simulink model "current_pi_model"  (R2023b)
settings: Solver=FixedStepDiscrete  StartTime=0.0  StopTime=current_pi_simcfg.stop_time  FixedStep=current_pi_simcfg.Ts_ctrl  RelTol=1e-3
values from neighbouring files (symbols this model uses):
  Kaw_id = 400.0    [current_pi_interface.sldd]
  Kaw_iq = 400.0    [current_pi_interface.sldd]
  Ki_id = 1072.4140625    [current_pi_interface.sldd]
  Ki_iq = 1072.4140625    [current_pi_interface.sldd]
  Kp_id = 1.3320353031158447    [current_pi_interface.sldd]
  Kp_iq = 1.3320353031158447    [current_pi_interface.sldd]
  VLimitRatio = 0.57700002193450928    [current_pi_interface.sldd]
undefined symbols (not defined in the file or in its folder): current_pi_simcfg, current_pi_test
settings Model: DataDictionary=current_pi_interface.sldd  Creator=user  LastModifiedBy=user
settings OptimizationCC: EnhancedBackFolding=on  PassReuseOutputArgsAs=Individual arguments  OptimizeBlockOrder=speed  DifferentSizesBufferReuse=on  OptimizationCustomize=off  EfficientTunableParamExpr=on
settings DebuggingCC: ParameterTunabilityLossMsg=error
settings HardwareCC: ProdBitPerPointer=32  ProdBitPerSizeT=32  ProdBitPerPtrDiffT=32  ProdLargestAtomicInteger=Long  ProdLargestAtomicFloat=Double  ProdWordSize=32  ProdHWDeviceType=ARM Compatible->ARM Cortex  TargetLargestAtomicInteger=Long  TargetLargestAtomicFloat=Double  TargetIntDivRoundTo=Zero  TargetEndianess=LittleEndian  TargetHWDeviceType=ARM Compatible->ARM Cortex  ProdEqTarget=off
settings SFSimCC: MATLABDynamicMemAlloc=off
settings RTWCC: Description=Embedded Coder  SystemTargetFile=ert.tlc  GenCodeOnly=on  TemplateMakefile=ert_default_tmf  GenerateReport=on
settings CodeAppCC: ForceParamTrailComments=on  IgnoreCustomStorageClasses=off  OperatorAnnotations=on  SimulinkDataObjDesc=on  SFDataObjDesc=on  InsertBlockDesc=on
settings ERTTargetCC: TargetLangStandard=C99 (ISO)  CodeInterfacePackaging=Reusable function  ERTCustomFileTemplate=example_file_process.tlc

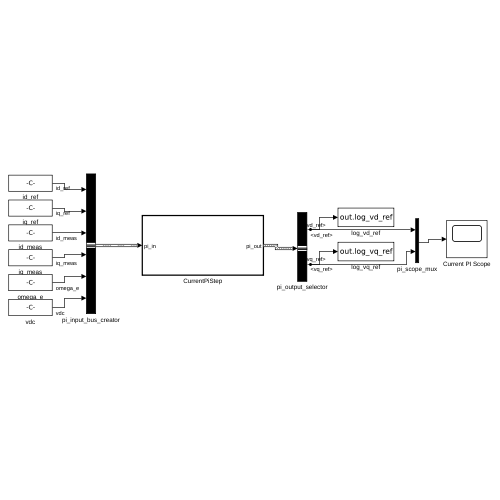
[thumbnail: Simulink's stored preview of the top-level diagram]
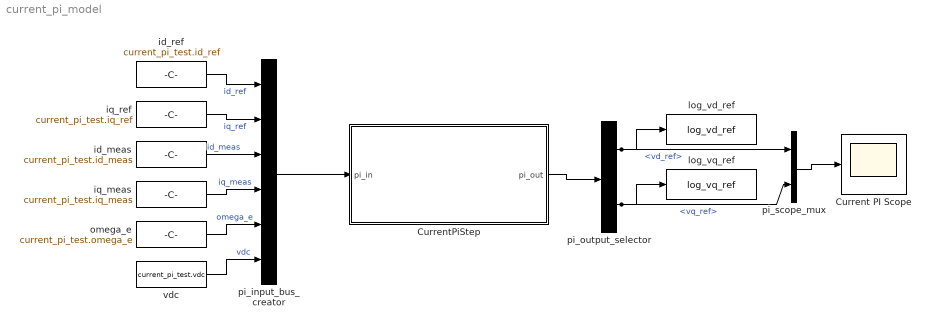
== system current_pi_model ==
  Current PI Scope : Scope
  CurrentPiStep : Subsystem  TreatAsAtomicUnit=on  RTWFcnName=CurrentPiStep  RTWFileName=CurrentPiStep
      settings: RTWFcnNameOpts=User specified  RTWFileNameOpts=User specified
  id_meas : Constant  Value=current_pi_test.id_meas  OutDataTypeStr=T_CurrentPiCurrent  SampleTime=current_pi_simcfg.Ts_ctrl
  id_ref : Constant  Value=current_pi_test.id_ref  OutDataTypeStr=T_CurrentPiCurrent  SampleTime=current_pi_simcfg.Ts_ctrl
  iq_meas : Constant  Value=current_pi_test.iq_meas  OutDataTypeStr=T_CurrentPiCurrent  SampleTime=current_pi_simcfg.Ts_ctrl
  iq_ref : Constant  Value=current_pi_test.iq_ref  OutDataTypeStr=T_CurrentPiCurrent  SampleTime=current_pi_simcfg.Ts_ctrl
  log_vd_ref : ToWorkspace  VariableName=log_vd_ref  SaveFormat=Timeseries  SampleTime=-1
  log_vq_ref : ToWorkspace  VariableName=log_vq_ref  SaveFormat=Timeseries  SampleTime=-1
  omega_e : Constant  Value=current_pi_test.omega_e  OutDataTypeStr=T_CurrentPiSpeed  SampleTime=current_pi_simcfg.Ts_ctrl
  pi_input_bus_creator : BusCreator  Inputs=6  OutDataTypeStr=Bus: current_pi_input_t  NonVirtualBus=on
  pi_output_selector : BusSelector  OutputSignals=vd_ref,vq_ref
  pi_scope_mux : Mux  Inputs=2
  vdc : Constant  Value=current_pi_test.vdc  OutDataTypeStr=T_CurrentPiVoltage  SampleTime=current_pi_simcfg.Ts_ctrl
  wires:
  id_ref/1 -> pi_input_bus_creator/1  "id_ref"
  iq_ref/1 -> pi_input_bus_creator/2  "iq_ref"
  id_meas/1 -> pi_input_bus_creator/3  "id_meas"
  iq_meas/1 -> pi_input_bus_creator/4  "iq_meas"
  omega_e/1 -> pi_input_bus_creator/5  "omega_e"
  vdc/1 -> pi_input_bus_creator/6  "vdc"
  pi_input_bus_creator/1 -> CurrentPiStep/1(pi_in)
  CurrentPiStep/1(pi_out) -> pi_output_selector/1
  pi_output_selector/1 -> log_vd_ref/1, pi_scope_mux/1  "<vd_ref>"
  pi_output_selector/2 -> log_vq_ref/1, pi_scope_mux/2  "<vq_ref>"
  pi_scope_mux/1 -> Current PI Scope/1

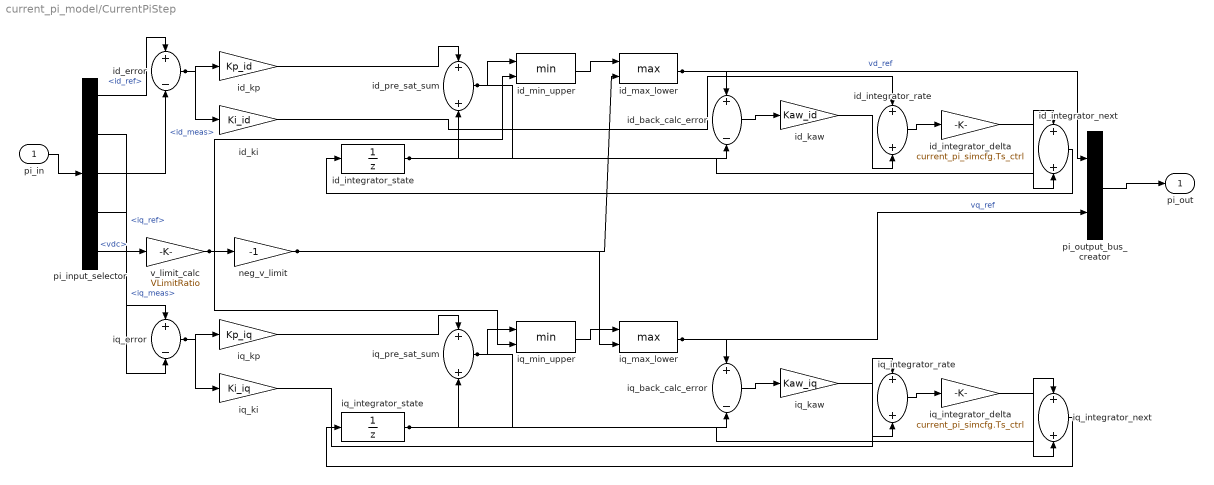
== system current_pi_model/CurrentPiStep ==
  pi_in : Inport  OutDataTypeStr=Bus: current_pi_input_t  BusOutputAsStruct=on
  id_back_calc_error : Sum  Inputs=+-  OutDataTypeStr=T_CurrentPiVoltage  AccumDataTypeStr=T_CurrentPiVoltage
  id_error : Sum  Inputs=+-  OutDataTypeStr=T_CurrentPiCurrent  AccumDataTypeStr=T_CurrentPiCurrent
  id_integrator_delta : Gain  Gain=current_pi_simcfg.Ts_ctrl  ParamDataTypeStr=T_CurrentPiFloat  OutDataTypeStr=T_CurrentPiVoltage
  id_integrator_next : Sum  OutDataTypeStr=T_CurrentPiVoltage  AccumDataTypeStr=T_CurrentPiVoltage
  id_integrator_rate : Sum  OutDataTypeStr=T_CurrentPiVoltage  AccumDataTypeStr=T_CurrentPiVoltage
  id_integrator_state : UnitDelay  SampleTime=current_pi_simcfg.Ts_ctrl  HasFrameUpgradeWarning=on
  id_kaw : Gain  Gain=Kaw_id  ParamDataTypeStr=T_CurrentPiGain  OutDataTypeStr=T_CurrentPiVoltage
  id_ki : Gain  Gain=Ki_id  ParamDataTypeStr=T_CurrentPiGain  OutDataTypeStr=T_CurrentPiVoltage
  id_kp : Gain  Gain=Kp_id  ParamDataTypeStr=T_CurrentPiGain  OutDataTypeStr=T_CurrentPiVoltage
  id_max_lower : MinMax  Function=max  Inputs=2
  id_min_upper : MinMax  Inputs=2
  id_pre_sat_sum : Sum  OutDataTypeStr=T_CurrentPiVoltage  AccumDataTypeStr=T_CurrentPiVoltage
  iq_back_calc_error : Sum  Inputs=+-  OutDataTypeStr=T_CurrentPiVoltage  AccumDataTypeStr=T_CurrentPiVoltage
  iq_error : Sum  Inputs=+-  OutDataTypeStr=T_CurrentPiCurrent  AccumDataTypeStr=T_CurrentPiCurrent
  iq_integrator_delta : Gain  Gain=current_pi_simcfg.Ts_ctrl  ParamDataTypeStr=T_CurrentPiFloat  OutDataTypeStr=T_CurrentPiVoltage
  iq_integrator_next : Sum  OutDataTypeStr=T_CurrentPiVoltage  AccumDataTypeStr=T_CurrentPiVoltage
  iq_integrator_rate : Sum  OutDataTypeStr=T_CurrentPiVoltage  AccumDataTypeStr=T_CurrentPiVoltage
  iq_integrator_state : UnitDelay  SampleTime=current_pi_simcfg.Ts_ctrl  HasFrameUpgradeWarning=on
  iq_kaw : Gain  Gain=Kaw_iq  ParamDataTypeStr=T_CurrentPiGain  OutDataTypeStr=T_CurrentPiVoltage
  iq_ki : Gain  Gain=Ki_iq  ParamDataTypeStr=T_CurrentPiGain  OutDataTypeStr=T_CurrentPiVoltage
  iq_kp : Gain  Gain=Kp_iq  ParamDataTypeStr=T_CurrentPiGain  OutDataTypeStr=T_CurrentPiVoltage
  iq_max_lower : MinMax  Function=max  Inputs=2
  iq_min_upper : MinMax  Inputs=2
  iq_pre_sat_sum : Sum  OutDataTypeStr=T_CurrentPiVoltage  AccumDataTypeStr=T_CurrentPiVoltage
  neg_v_limit : Gain  Gain=-1  ParamDataTypeStr=T_CurrentPiFloat  OutDataTypeStr=T_CurrentPiVoltage
  pi_input_selector : BusSelector  OutputSignals=id_ref,iq_ref,id_meas,iq_meas,vdc
  pi_output_bus_creator : BusCreator  Inputs=2  OutDataTypeStr=Bus: current_pi_output_t  NonVirtualBus=on
  v_limit_calc : Gain  Gain=VLimitRatio  ParamDataTypeStr=T_CurrentPiGain  OutDataTypeStr=T_CurrentPiVoltage
  pi_out : Outport  OutDataTypeStr=Bus: current_pi_output_t
  wires:
  pi_in/1 -> pi_input_selector/1
  pi_input_selector/5 -> v_limit_calc/1  "<vdc>"
  v_limit_calc/1 -> neg_v_limit/1, id_min_upper/2, iq_min_upper/2
  pi_input_selector/1 -> id_error/1  "<id_ref>"
  pi_input_selector/3 -> id_error/2  "<id_meas>"
  id_error/1 -> id_kp/1, id_ki/1
  id_kp/1 -> id_pre_sat_sum/1
  id_integrator_state/1 -> id_pre_sat_sum/2, id_integrator_next/1
  id_pre_sat_sum/1 -> id_min_upper/1, id_back_calc_error/2
  id_min_upper/1 -> id_max_lower/1
  neg_v_limit/1 -> id_max_lower/2, iq_max_lower/2
  id_max_lower/1 -> id_back_calc_error/1, pi_output_bus_creator/1  "vd_ref"
  id_back_calc_error/1 -> id_kaw/1
  id_ki/1 -> id_integrator_rate/1
  id_kaw/1 -> id_integrator_rate/2
  id_integrator_rate/1 -> id_integrator_delta/1
  id_integrator_delta/1 -> id_integrator_next/2
  id_integrator_next/1 -> id_integrator_state/1
  pi_input_selector/2 -> iq_error/1  "<iq_ref>"
  pi_input_selector/4 -> iq_error/2  "<iq_meas>"
  iq_error/1 -> iq_kp/1, iq_ki/1
  iq_kp/1 -> iq_pre_sat_sum/1
  iq_integrator_state/1 -> iq_pre_sat_sum/2, iq_integrator_next/1
  iq_pre_sat_sum/1 -> iq_min_upper/1, iq_back_calc_error/2
  iq_min_upper/1 -> iq_max_lower/1
  iq_max_lower/1 -> iq_back_calc_error/1, pi_output_bus_creator/2  "vq_ref"
  iq_back_calc_error/1 -> iq_kaw/1
  iq_ki/1 -> iq_integrator_rate/1
  iq_kaw/1 -> iq_integrator_rate/2
  iq_integrator_rate/1 -> iq_integrator_delta/1
  iq_integrator_delta/1 -> iq_integrator_next/2
  iq_integrator_next/1 -> iq_integrator_state/1
  pi_output_bus_creator/1 -> pi_out/1
